simulink model "Retro_Edo_3_COpt"  (Simulink 8.6)
settings: Solver=ode45  StartTime=0.0  StopTime=10.0  RelTol=1e-3
values from neighbouring files (symbols this model uses):
  A = [0 1 0 ... (first row only)    [COpt.m]    (also in Ob_Edo.m; Retro_Edo 2.m)
  b = [0; 0; 1]    [COpt.m]    (also in Ob_Edo.m; Retro_Edo 2.m)
  Id = eye(3)    [COpt.m]    (also in Ob_Edo.m; Retro_Edo 2.m)
  r = 1/10    (= 0.1)    [COpt.m]
  vcero = zeros(3,1)    [COpt.m]    (also in Ob_Edo.m; Retro_Edo 2.m)
  x0 = [1; 0; 0]    [COpt.m]    (also in Ob_Edo.m; Retro_Edo 2.m)
settings Model: Creator=Tlakatl  LastModifiedBy=Tlayekanketl
settings DebuggingCC: SolverPrmCheckMsg=none  FcnCallInpInsideContextMsg=EnableAllAsWarning
settings ConfigComp: CovSFcnEnable=off

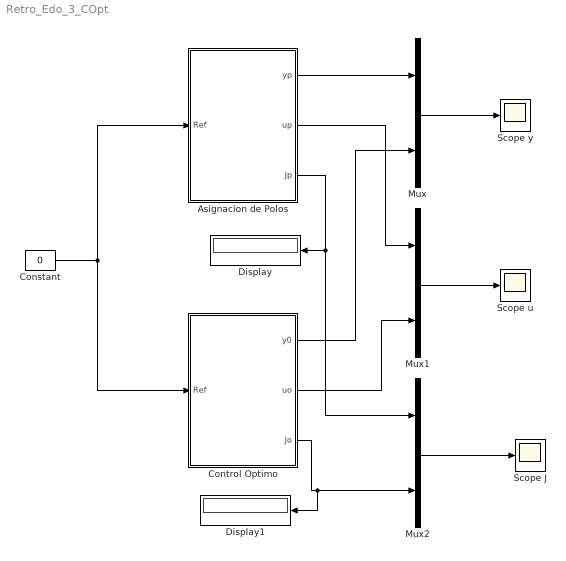
== system Retro_Edo_3_COpt ==
  Asignacion de Polos : Subsystem
  Constant : Constant  Value=0
  Control Optimo : Subsystem
  Display : Display
  Display1 : Display
  Mux : Mux  Inputs=2
  Mux1 : Mux  Inputs=2
  Mux2 : Mux  Inputs=2
  Scope J : Scope
  Scope u : Scope
  Scope y : Scope
  wires:
  Constant/1 -> Control Optimo/1(Ref), Asignacion de Polos/1(Ref)
  Asignacion de Polos/1(yp) -> Mux/1
  Control Optimo/1(y0) -> Mux/2
  Mux/1 -> Scope y/1
  Control Optimo/2(uo) -> Mux1/2
  Asignacion de Polos/2(up) -> Mux1/1
  Mux1/1 -> Scope u/1
  Mux2/1 -> Scope J/1
  Control Optimo/3(Jo) -> Display1/1, Mux2/2
  Asignacion de Polos/3(Jp) -> Display/1, Mux2/1

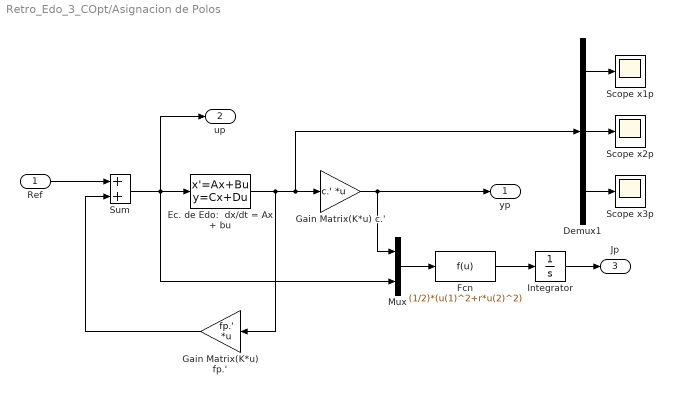
== system Retro_Edo_3_COpt/Asignacion de Polos ==
  Ref : Inport
  Demux1 : Demux  Outputs=3
  Ec. de Edo:  dx/dt = Ax + bu : StateSpace  A=A  B=b  C=Id  D=vcero  X0=x0
  Fcn : Fcn  Expr=(1/2)*(u(1)^2+r*u(2)^2)
  Gain Matrix(K*u) c.' : Gain  Gain=c.'  Multiplication=Matrix(K*u) (u vector)
  Gain Matrix(K*u) fp.' : Gain  Gain=fp.'  Multiplication=Matrix(K*u) (u vector)
  Integrator : Integrator
  Mux : Mux  Inputs=2
  Scope x1p : Scope
  Scope x2p : Scope
  Scope x3p : Scope
  Sum : Sum
  yp : Outport
  up : Outport  Port=2
  Jp : Outport  Port=3
  wires:
  Sum/1 -> Mux/2, up/1, Ec. de Edo:  dx/dt = Ax + bu/1
  Ec. de Edo:  dx/dt = Ax + bu/1 -> Gain Matrix(K*u) fp.'/1, Demux1/1, Gain Matrix(K*u) c.'/1
  Gain Matrix(K*u) fp.'/1 -> Sum/2
  Ref/1 -> Sum/1
  Gain Matrix(K*u) c.'/1 -> Mux/1, yp/1
  Mux/1 -> Fcn/1
  Fcn/1 -> Integrator/1
  Integrator/1 -> Jp/1
  Demux1/3 -> Scope x3p/1
  Demux1/2 -> Scope x2p/1
  Demux1/1 -> Scope x1p/1

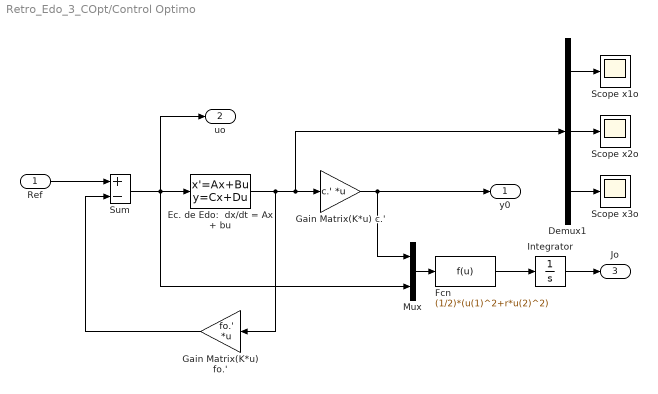
== system Retro_Edo_3_COpt/Control Optimo ==
  Ref : Inport
  Demux1 : Demux  Outputs=3
  Ec. de Edo:  dx/dt = Ax + bu : StateSpace  A=A  B=b  C=Id  D=vcero  X0=x0
  Fcn : Fcn  Expr=(1/2)*(u(1)^2+r*u(2)^2)
  Gain Matrix(K*u) c.' : Gain  Gain=c.'  Multiplication=Matrix(K*u) (u vector)
  Gain Matrix(K*u) fo.' : Gain  Gain=fo.'  Multiplication=Matrix(K*u) (u vector)
  Integrator : Integrator
  Mux : Mux  Inputs=2
  Scope x1o : Scope
  Scope x2o : Scope
  Scope x3o : Scope
  Sum : Sum  Inputs=+-
  y0 : Outport
  uo : Outport  Port=2
  Jo : Outport  Port=3
  wires:
  Sum/1 -> Mux/2, uo/1, Ec. de Edo:  dx/dt = Ax + bu/1
  Ec. de Edo:  dx/dt = Ax + bu/1 -> Gain Matrix(K*u) fo.'/1, Demux1/1, Gain Matrix(K*u) c.'/1
  Gain Matrix(K*u) fo.'/1 -> Sum/2
  Ref/1 -> Sum/1
  Gain Matrix(K*u) c.'/1 -> Mux/1, y0/1
  Mux/1 -> Fcn/1
  Fcn/1 -> Integrator/1
  Integrator/1 -> Jo/1
  Demux1/3 -> Scope x3o/1
  Demux1/2 -> Scope x2o/1
  Demux1/1 -> Scope x1o/1
